simulink model "simulate_ackermann"  (R2022b)
settings: Solver=FixedStepAuto  StartTime=0.0  StopTime=1  FixedStep=0.01  RelTol=1e-3
libraries: robotmobilelib x1
settings Model: Creator=Miakho  LastModifiedBy=Miakho

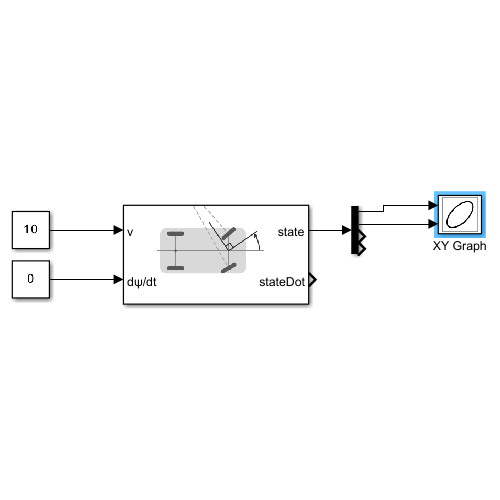
[thumbnail: Simulink's stored preview of the top-level diagram]
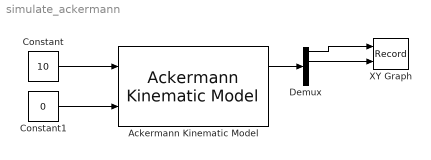
== system simulate_ackermann ==
  Ackermann Kinematic Model : robotmobilelib/Ackermann Kinematic Model  WheelBase=2.908  VehicleSpeedRange=[-inf inf]  MaxSteeringAngle=pi/6  InitialState=[0; 0; 0; 0.1]  SimulateUsing=Interpreted execution
  Constant : Constant  Value=10
  Constant1 : Constant  Value=0
  Demux : Demux
  XY Graph : Record  FileSettingsInternal="{\"entries\":[{\"content\":{\"excelSettings\":{\"content\":{},\"type\":\"Streamout.ExcelSettings\"}},\"type\":\"Streamout.FileSettingStorage\",\"uuid\":\"6fbf6788-41ce-44ce-af92-e7636d68e526\"}],\"packageUris\":[\"http://schema.mathworks.com/mf0/streamout_blocks/R2020a\"],\"version\":\"1.0\"}"  Layout=[1 1]  SignalsInternal="{\"entries\":[{\"content\":{\"signals\":[{\"content\":{\"blockPath\":[\"simulate_ackermann/XY Graph\"],\"channel\":[],\"dimensions\":[1],\"domain\":\"simulate_ackermann/XY Graph\",\"lineColor\":\"#a2142f\",\"plots\":[1],\"port\":1,\"sid\":[\"\"],\"signalID\":284,\"signalName\":\"Demux:1\"},\"type\":\"RecordBlkView.Signal\",\"uuid\":\"f871c00e-4c25-43e4-b121-f0c9d786126c\"},{\"content\":{\"blockPath\":[\"simulate_ackermann/XY Graph\"],\"channel\":[],\"dimensions\":[1],\"domain\":\"simulate_ackermann/XY Graph\",\"lineColor\":\"#139fff\",\"plots\":[1],\"port\":2,\"sid\":[\"\"],\"signalID\":288,\"signalName\":\"Demux:2\"},\"type\":\"RecordBlkView.Signal\",\"uuid\":\"1630c0b0-2877-4686-929f-08f0074512a3\"}]},\"type\":\"RecordBlkView.InputSignals\",\"uuid\":\"edca76d9-994f-4855-b887-b0e67c18a998\"}],\"packageUris\":[\"http://schema.mathworks.com/mf0/streamout_blocks/R2020a\"],\"version\":\"1.0\"}"  VisualizationBindings="{\"xyplotplugin\":{\"info\":[{\"series\":[{\"bindingParametersList\":[{\"parameter\":\"X-Axis\",\"signalID\":284,\"signalName\":\"Demux:1\"},{\"parameter\":\"Y-Axis\",\"signalID\":288,\"signalName\":\"Demux:2\"}],\"seriesID\":37882}],\"subplotID\":1}]}}"  CompatibilityTag=XY
  wires:
  Constant/1 -> Ackermann Kinematic Model/1
  Constant1/1 -> Ackermann Kinematic Model/2
  Ackermann Kinematic Model/1 -> Demux/1
  Demux/1 -> XY Graph/1
  Demux/2 -> XY Graph/2
